simulink model "Scenario"  (Simulink 7.7)
settings: Solver=ode45  StartTime=0.0  StopTime=10.0  RelTol=1e-3
undefined symbols (not defined in the file): sigbuilder_block
libraries: simulink x4, instrumentlib x4, utility x1, dspnetwork x1
settings Model: Creator=Zsolt  LastModifiedBy=meta
settings HardwareCC: TargetIntDivRoundTo=Zero  TargetEndianess=LittleEndian  TargetHWDeviceType=MATLAB Host  ProdEqTarget=off
settings RTWCC: SystemTargetFile=rsim.tlc  TemplateMakefile=rsim_default_tmf  Description=Rapid Simulation Target  ProcessScript=rsim_make_rtw_hook
settings RSimTargetCC: TargetFunctionLibrary=ANSI_C  ERTMultiwordTypeDef=System defined  FunctionExecutionProfile=off  CodeExecutionProfiling=off  ERTCodeCoverageTool=None  ERTMultiwordLength=256  IsPILTarget=off  EnableShiftOperators=on  PortableWordSizes=off

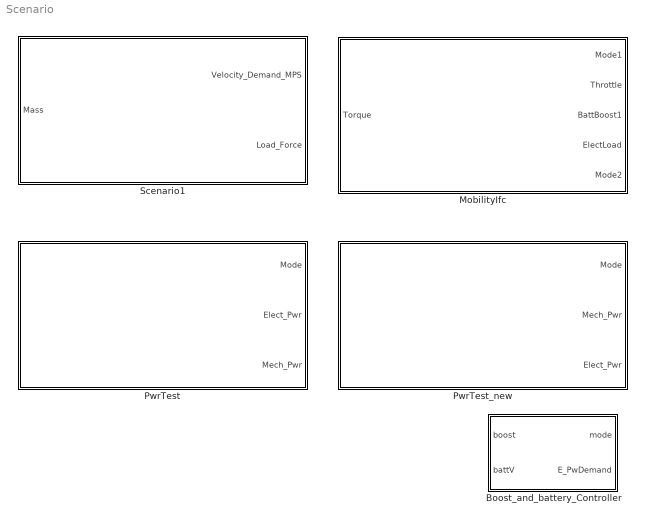
== system Scenario ==
  Boost_and_battery_Controller : Stateflow chart  TreatAsAtomicUnit=on
  MobilityIfc : Subsystem
  PwrTest : Subsystem
  PwrTest_new : Subsystem
  Scenario1 : Subsystem

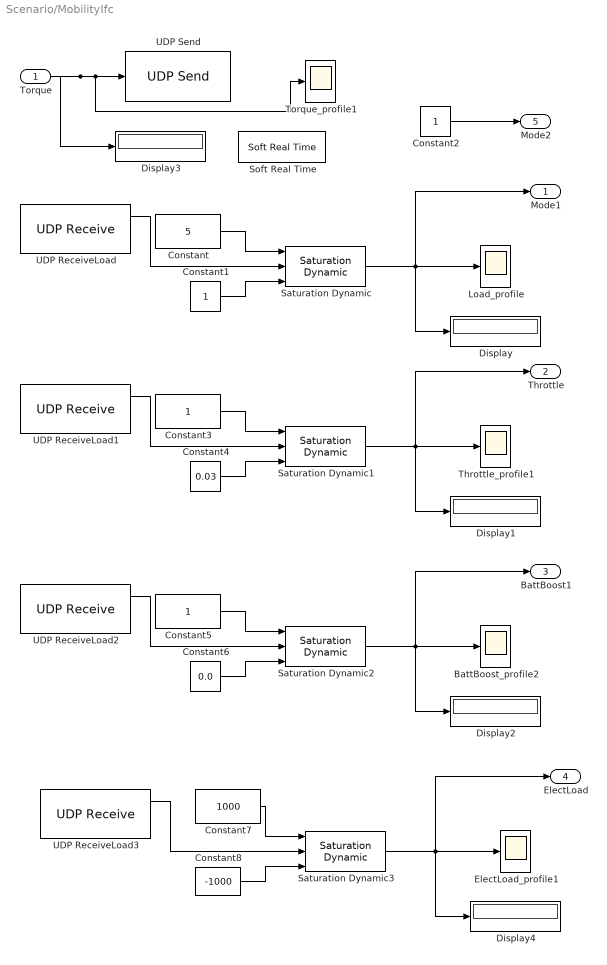
== system Scenario/MobilityIfc ==
  Torque : Inport
  BattBoost_profile2 : Scope
      settings: TimeRange=500  YMin=0  YMax=150000  SaveName=ScopeData3
  Constant : Constant  Value=5
  Constant{1..3,5} (4 alike) : Constant
  Constant4 : Constant  Value=0.03
  Constant6 : Constant  Value=0.0
  Constant7 : Constant  Value=1000
  Constant8 : Constant  Value=-1000
  Display{,1..4} (5 alike) : Display
  ElectLoad_profile1 : Scope
      settings: TimeRange=500  YMin=0  YMax=150000  SaveName=ScopeData5
  Load_profile : Scope
      settings: TimeRange=500  YMin=0  YMax=150000
  Saturation Dynamic{,1..3} (4 alike) : simulink/Discontinuities/Saturation Dynamic  SystemSampleTime=-1  OutMin=[]  OutMax=[]  OutDataTypeStr=Inherit: Same as second input  OutDataType=fixdt(1, 16)  OutScaling=2^-10  DoSatur=off
  Soft Real Time : utility/Soft Real Time  x=1
  Throttle_profile1 : Scope
      settings: TimeRange=500  YMin=0  YMax=150000
  Torque_profile1 : Scope
      settings: TimeRange=100  YMin=0  YMax=150000  SaveName=ScopeData4
  UDP ReceiveLoad : instrumentlib/UDP Receive  Host=localhost  Port=9090  LocalPort=8090  DataSize=[1 1]  EnableBlockingMode=off  Timeout=10  SampleTime=0.08  DataType=double  ByteOrder=LittleEndian
  UDP ReceiveLoad1 : instrumentlib/UDP Receive  Host=localhost  Port=9090  LocalPort=8092  DataSize=[1 1]  EnableBlockingMode=off  Timeout=10  SampleTime=0.08  DataType=double  ByteOrder=LittleEndian
  UDP ReceiveLoad2 : instrumentlib/UDP Receive  Host=localhost  Port=9090  LocalPort=8093  DataSize=[1 1]  EnableBlockingMode=off  Timeout=10  SampleTime=0.08  DataType=double  ByteOrder=LittleEndian
  UDP ReceiveLoad3 : instrumentlib/UDP Receive  Host=localhost  Port=9090  LocalPort=8098  DataSize=[1 1]  EnableBlockingMode=off  Timeout=10  SampleTime=0.08  DataType=double  ByteOrder=LittleEndian
  UDP Send : dspnetwork/UDP Send  remoteURL='127.0.0.1'  remotePort=8094  localURL='0.0.0.0'  localPortSource=Automatically determine  localPort=-1  sampletime=-1  separateLengthPort=0
  Mode1 : Outport
  Throttle : Outport  Port=2
  BattBoost1 : Outport  Port=3
  ElectLoad : Outport  Port=4
  Mode2 : Outport  Port=5
  wires:
  Constant/1 -> Saturation Dynamic/1
  Constant1/1 -> Saturation Dynamic/3
  Saturation Dynamic/1 -> Load_profile/1, Display/1, Mode1/1
  UDP ReceiveLoad/1 -> Saturation Dynamic/2
  Constant2/1 -> Mode2/1
  Constant3/1 -> Saturation Dynamic1/1
  Constant4/1 -> Saturation Dynamic1/3
  Saturation Dynamic1/1 -> Throttle_profile1/1, Display1/1, Throttle/1
  UDP ReceiveLoad1/1 -> Saturation Dynamic1/2
  Constant5/1 -> Saturation Dynamic2/1
  Constant6/1 -> Saturation Dynamic2/3
  Saturation Dynamic2/1 -> BattBoost_profile2/1, Display2/1, BattBoost1/1
  UDP ReceiveLoad2/1 -> Saturation Dynamic2/2
  Torque/1 -> UDP Send/1, Torque_profile1/1, Display3/1
  Constant7/1 -> Saturation Dynamic3/1
  Constant8/1 -> Saturation Dynamic3/3
  Saturation Dynamic3/1 -> ElectLoad_profile1/1, Display4/1, ElectLoad/1
  UDP ReceiveLoad3/1 -> Saturation Dynamic3/2

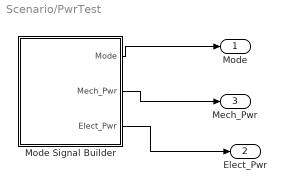
== system Scenario/PwrTest ==
  Mode Signal Builder : Subsystem  Tag=STV Subsys  LoadFcn=sigbuilder_block('load');  StartFcn=sigbuilder_block('start');  StopFcn=sigbuilder_block('stop');  ClipboardFcn=sigbuilder_block('clipboard');  mask(Sigbuilder block){}
      mask help: Create and generate interchangeable groups of signals whose waveforms are piecewise linear.
      mask init:
      | if ~strcmp(get_param(bdroot(gcbh),'SimulationStatus'),'stopped') tuvar = sigbuilder_block('maskInit'); end
      settings: CopyFcn=sigbuilder_block('copy');  DeleteFcn=sigbuilder_block('delete');  ModelCloseFcn=sigbuilder_block('modelClose');  PreSaveFcn=sigbuilder_block('preSave');  NameChangeFcn=sigbuilder_block('namechange');  OpenFcn=sigbuilder_block('open',[215.25 65.25 852.75 489.75 ]);  CloseFcn=sigbuilder_block('close');
      mask Display: plot(0,0,100,100,[10,10,40,40,10],[80,20,20,80,80],[40,10],[50,50], [40,27,10],[65,72,56],[40,25,25,10],[28,28,43,43]);
  Mode : Outport
  Elect_Pwr : Outport  Port=2
  Mech_Pwr : Outport  Port=3
  wires:
  Mode Signal Builder/1(Mode) -> Mode/1
  Mode Signal Builder/2(Mech_Pwr) -> Mech_Pwr/1
  Mode Signal Builder/3(Elect_Pwr) -> Elect_Pwr/1

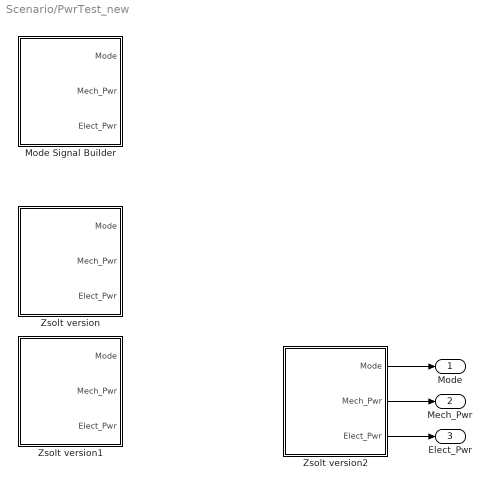
== system Scenario/PwrTest_new ==
  Mode Signal Builder : Subsystem  Tag=STV Subsys  LoadFcn=sigbuilder_block('load');  StartFcn=sigbuilder_block('start');  StopFcn=sigbuilder_block('stop');  ClipboardFcn=sigbuilder_block('clipboard');  mask(Sigbuilder block){}
      mask help: Create and generate interchangeable groups of signals whose waveforms are piecewise linear.
      mask init:
      | if ~strcmp(get_param(bdroot(gcbh),'SimulationStatus'),'stopped') tuvar = sigbuilder_block('maskInit'); end
      settings: CopyFcn=sigbuilder_block('copy');  DeleteFcn=sigbuilder_block('delete');  ModelCloseFcn=sigbuilder_block('modelClose');  PreSaveFcn=sigbuilder_block('preSave');  NameChangeFcn=sigbuilder_block('namechange');  OpenFcn=sigbuilder_block('open',[215.25 65.25 852.75 489.75 ]);  CloseFcn=sigbuilder_block('close');
      mask Display: plot(0,0,100,100,[10,10,40,40,10],[80,20,20,80,80],[40,10],[50,50], [40,27,10],[65,72,56],[40,25,25,10],[28,28,43,43]);
  Zsolt version : Subsystem  Tag=STV Subsys  LoadFcn=sigbuilder_block('load');  StartFcn=sigbuilder_block('start');  StopFcn=sigbuilder_block('stop');  ClipboardFcn=sigbuilder_block('clipboard');  mask(Sigbuilder block){}
      mask help: Create and generate interchangeable groups of signals whose waveforms are piecewise linear.
      mask init:
      | if ~strcmp(get_param(bdroot(gcbh),'SimulationStatus'),'stopped') tuvar = sigbuilder_block('maskInit'); end
      settings: CopyFcn=sigbuilder_block('copy');  DeleteFcn=sigbuilder_block('delete');  ModelCloseFcn=sigbuilder_block('modelClose');  PreSaveFcn=sigbuilder_block('preSave');  NameChangeFcn=sigbuilder_block('namechange');  OpenFcn=sigbuilder_block('open',[9 35.25 852.75 281.25 ]);  CloseFcn=sigbuilder_block('close');
      mask Display: plot(0,0,100,100,[10,10,40,40,10],[80,20,20,80,80],[40,10],[50,50], [40,27,10],[65,72,56],[40,25,25,10],[28,28,43,43]);
  Zsolt version1 : Subsystem  Tag=STV Subsys  LoadFcn=sigbuilder_block('load');  StartFcn=sigbuilder_block('start');  StopFcn=sigbuilder_block('stop');  ClipboardFcn=sigbuilder_block('clipboard');  mask(Sigbuilder block){}
      mask help: Create and generate interchangeable groups of signals whose waveforms are piecewise linear.
      mask init:
      | if ~strcmp(get_param(bdroot(gcbh),'SimulationStatus'),'stopped') tuvar = sigbuilder_block('maskInit'); end
      settings: CopyFcn=sigbuilder_block('copy');  DeleteFcn=sigbuilder_block('delete');  ModelCloseFcn=sigbuilder_block('modelClose');  PreSaveFcn=sigbuilder_block('preSave');  NameChangeFcn=sigbuilder_block('namechange');  OpenFcn=sigbuilder_block('open',[9 35.25 852.75 281.25 ]);  CloseFcn=sigbuilder_block('close');
      mask Display: plot(0,0,100,100,[10,10,40,40,10],[80,20,20,80,80],[40,10],[50,50], [40,27,10],[65,72,56],[40,25,25,10],[28,28,43,43]);
  Zsolt version2 : Subsystem  Tag=STV Subsys  LoadFcn=sigbuilder_block('load');  StartFcn=sigbuilder_block('start');  StopFcn=sigbuilder_block('stop');  ClipboardFcn=sigbuilder_block('clipboard');  mask(Sigbuilder block){}
      mask help: Create and generate interchangeable groups of signals whose waveforms are piecewise linear.
      mask init:
      | if ~strcmp(get_param(bdroot(gcbh),'SimulationStatus'),'stopped') tuvar = sigbuilder_block('maskInit'); end
      settings: CopyFcn=sigbuilder_block('copy');  DeleteFcn=sigbuilder_block('delete');  ModelCloseFcn=sigbuilder_block('modelClose');  PreSaveFcn=sigbuilder_block('preSave');  NameChangeFcn=sigbuilder_block('namechange');  OpenFcn=sigbuilder_block('open',[8.25 -66 852.75 246 ]);  CloseFcn=sigbuilder_block('close');
      mask Display: plot(0,0,100,100,[10,10,40,40,10],[80,20,20,80,80],[40,10],[50,50], [40,27,10],[65,72,56],[40,25,25,10],[28,28,43,43]);
  Mode : Outport
  Mech_Pwr : Outport  Port=2
  Elect_Pwr : Outport  Port=3
  wires:
  Zsolt version2/1(Mode) -> Mode/1
  Zsolt version2/2(Mech_Pwr) -> Mech_Pwr/1
  Zsolt version2/3(Elect_Pwr) -> Elect_Pwr/1

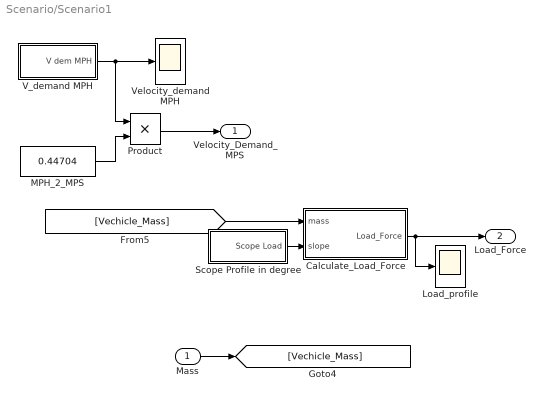
== system Scenario/Scenario1 ==
  Mass : Inport
  Calculate_Load_Force : Subsystem
  Load_profile : Scope
      settings: TimeRange=500  YMin=0  YMax=100000  SaveName=ScopeData7
  MPH_2_MPS : Constant  Value=0.44704
  Product : Product  RndMeth=Zero
  Scope Profile in degree : Subsystem  Tag=STV Subsys  LoadFcn=sigbuilder_block('load');  StartFcn=sigbuilder_block('start');  StopFcn=sigbuilder_block('stop');  ClipboardFcn=sigbuilder_block('clipboard');  mask(Sigbuilder block){}
      mask help: Create and generate interchangeable groups of signals whose waveforms are piecewise linear.
      mask init:
      | if ~strcmp(get_param(bdroot(gcbh),'SimulationStatus'),'stopped') tuvar = sigbuilder_block('maskInit'); end
      settings: CopyFcn=sigbuilder_block('copy');  DeleteFcn=sigbuilder_block('delete');  ModelCloseFcn=sigbuilder_block('modelClose');  PreSaveFcn=sigbuilder_block('preSave');  NameChangeFcn=sigbuilder_block('namechange');  OpenFcn=sigbuilder_block('open',[879 269.25 550.5 386.25 ]);  CloseFcn=sigbuilder_block('close');
      mask Display: plot(0,0,100,100,[10,10,40,40,10],[80,20,20,80,80],[40,10],[50,50], [40,27,10],[65,72,56],[40,25,25,10],[28,28,43,43]);
  V_demand MPH : Subsystem  Tag=STV Subsys  LoadFcn=sigbuilder_block('load');  StartFcn=sigbuilder_block('start');  StopFcn=sigbuilder_block('stop');  ClipboardFcn=sigbuilder_block('clipboard');  mask(Sigbuilder block){}
      mask help: Create and generate interchangeable groups of signals whose waveforms are piecewise linear.
      mask init:
      | if ~strcmp(get_param(bdroot(gcbh),'SimulationStatus'),'stopped') tuvar = sigbuilder_block('maskInit'); end
      settings: CopyFcn=sigbuilder_block('copy');  DeleteFcn=sigbuilder_block('delete');  ModelCloseFcn=sigbuilder_block('modelClose');  PreSaveFcn=sigbuilder_block('preSave');  NameChangeFcn=sigbuilder_block('namechange');  OpenFcn=sigbuilder_block('open',[827.25 153 606.75 301.5 ]);  CloseFcn=sigbuilder_block('close');
      mask Display: plot(0,0,100,100,[10,10,40,40,10],[80,20,20,80,80],[40,10],[50,50], [40,27,10],[65,72,56],[40,25,25,10],[28,28,43,43]);
  Velocity_demand MPH : Scope
      settings: TimeRange=500  YMin=0  YMax=60  SaveName=ScopeData2
  Velocity_Demand_MPS : Outport
  Load_Force : Outport  Port=2
  wires:
  MPH_2_MPS/1 -> Product/2
  V_demand MPH/1(V dem MPH) -> Product/1, Velocity_demand MPH/1
  Product/1 -> Velocity_Demand_MPS/1
  Calculate_Load_Force/1(Load_Force) -> Load_profile/1, Load_Force/1
  Scope Profile in degree/1(Scope Load) -> Calculate_Load_Force/2(slope)
  [Vechicle_Mass] -> Calculate_Load_Force/1(mass)
  Mass/1 -> [Vechicle_Mass]

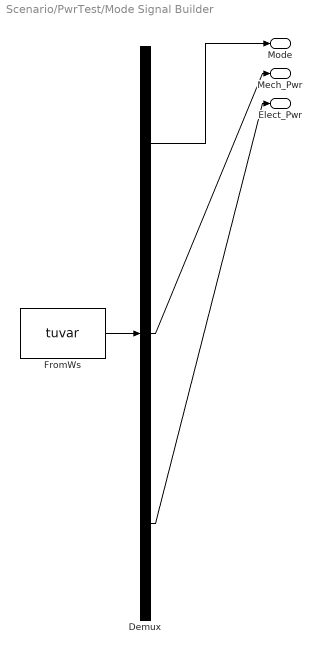
== system Scenario/PwrTest/Mode Signal Builder ==
  Demux : Demux  Tag=STV Demux  Outputs=3
  FromWs : FromWorkspace  Tag=STV FromWs  VariableName=tuvar  SampleTime=0  SigBuilderData=DataTag0  VnvData=DataTag1
      SigBuilderData=|
      | common.afterFinalStr = 'Extrapolate'
      | common.sampleTime = 0
      | dataSet.timeRange = [0 1000]
      | dataSet.name = 'Group 1'
      | sbobj.Groups.Name = 'Group 1'
      | sbobj.Groups.Signals(1).Name = 'Mode'
      | sbobj.Groups.Signals(1).XData = [0 62 62 398 1000]
      | sbobj.Groups.Signals(1).YData = [1 1 0 0 0]
      | sbobj.Groups.Signals(2).Name = 'Mech_Pwr'
      | sbobj.Groups.Signals(2).XData = [0 16 16 239 239 1000]
      | sbobj.Groups.Signals(2).YData = [0.58 0.58 0.24 0.24 0.44 0.44]
      | sbobj.Groups.Signals(3).Name = 'Elect_Pwr'
      | sbobj.Groups.Signals(3).XData = [0 16 16 44 44 60 60 81 81 1000]
      | sbobj.Groups.Signals(3).YData = [37 37 -32.5 -32.5 -0.5 -0.5 -1 -1 -1 -1]
      | sbobj.Groups.TimeRange = [0 1000]
  Mode : Outport  Tag=STV Outport
  Mech_Pwr : Outport  Tag=STV Outport  Port=2
  Elect_Pwr : Outport  Tag=STV Outport  Port=3
  wires:
  Demux/1 -> Mode/1
  FromWs/1 -> Demux/1
  Demux/2 -> Mech_Pwr/1
  Demux/3 -> Elect_Pwr/1

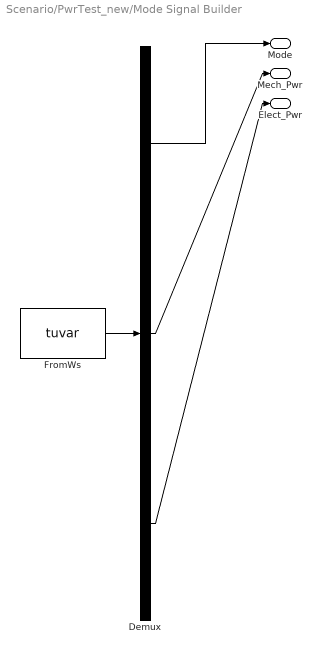
== system Scenario/PwrTest_new/Mode Signal Builder ==
  Demux : Demux  Tag=STV Demux  Outputs=3
  FromWs : FromWorkspace  Tag=STV FromWs  VariableName=tuvar  SampleTime=0  SigBuilderData=DataTag2  VnvData=DataTag3
      SigBuilderData=|
      | common.afterFinalStr = 'Extrapolate'
      | common.sampleTime = 0
      | dataSet.timeRange = [0 1000]
      | dataSet.name = 'Group 1'
      | sbobj.Groups.Name = 'Group 1'
      | sbobj.Groups.Signals(1).Name = 'Mode'
      | sbobj.Groups.Signals(1).XData = [0 62 62 398 1000]
      | sbobj.Groups.Signals(1).YData = [1 1 0 0 0]
      | sbobj.Groups.Signals(2).Name = 'Mech_Pwr'
      | sbobj.Groups.Signals(2).XData = [0 16 16 239 239 1000]
      | sbobj.Groups.Signals(2).YData = [0.58 0.58 0.24 0.24 0.44 0.44]
      | sbobj.Groups.Signals(3).Name = 'Elect_Pwr'
      | sbobj.Groups.Signals(3).XData = [0 16 16 44 44 60 60 81 81 1000]
      | sbobj.Groups.Signals(3).YData = [37 37 -32.5 -32.5 -0.5 -0.5 -1 -1 -1 -1]
      | sbobj.Groups.TimeRange = [0 1000]
  Mode : Outport  Tag=STV Outport
  Mech_Pwr : Outport  Tag=STV Outport  Port=2
  Elect_Pwr : Outport  Tag=STV Outport  Port=3
  wires:
  Demux/3 -> Elect_Pwr/1
  Demux/2 -> Mech_Pwr/1
  FromWs/1 -> Demux/1
  Demux/1 -> Mode/1

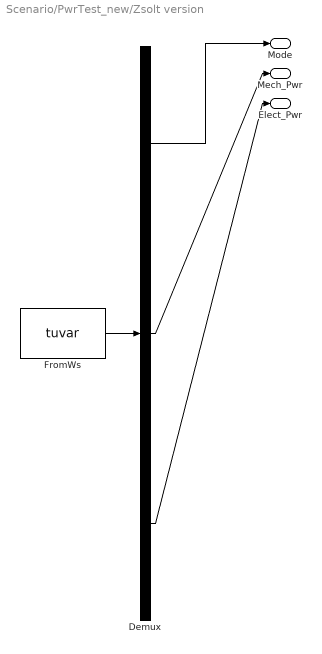
== system Scenario/PwrTest_new/Zsolt version ==
  Demux : Demux  Tag=STV Demux  Outputs=3
  FromWs : FromWorkspace  Tag=STV FromWs  VariableName=tuvar  SampleTime=0  SigBuilderData=DataTag4  VnvData=DataTag5
      SigBuilderData=|
      | common.afterFinalStr = 'Extrapolate'
      | common.sampleTime = 0
      | dataSet.timeRange = [0 100]
      | dataSet.name = 'Group 1'
      | sbobj.Groups.Name = 'Group 1'
      | sbobj.Groups.Signals(1).Name = 'Mode'
      | sbobj.Groups.Signals(1).XData = [0 62 62 100]
      | sbobj.Groups.Signals(1).YData = [1 1 0 0]
      | sbobj.Groups.Signals(2).Name = 'Mech_Pwr'
      | sbobj.Groups.Signals(2).XData = [0 24.7 100]
      | sbobj.Groups.Signals(2).YData = [0.68 0.68 0.24]
      | sbobj.Groups.Signals(3).Name = 'Elect_Pwr'
      | sbobj.Groups.Signals(3).XData = [0 2 2 25.6 25.6 28 28 100]
      | sbobj.Groups.Signals(3).YData = [-208 -208 -288 -284 -212 -212 -202 -202]
      | sbobj.Groups.TimeRange = [0 100]
  Mode : Outport  Tag=STV Outport
  Mech_Pwr : Outport  Tag=STV Outport  Port=2
  Elect_Pwr : Outport  Tag=STV Outport  Port=3
  wires:
  Demux/3 -> Elect_Pwr/1
  Demux/2 -> Mech_Pwr/1
  FromWs/1 -> Demux/1
  Demux/1 -> Mode/1

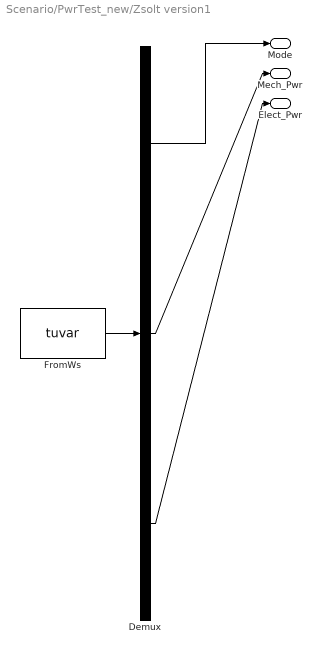
== system Scenario/PwrTest_new/Zsolt version1 ==
  Demux : Demux  Tag=STV Demux  Outputs=3
  FromWs : FromWorkspace  Tag=STV FromWs  VariableName=tuvar  SampleTime=0  SigBuilderData=DataTag6  VnvData=DataTag7
      SigBuilderData=|
      | common.afterFinalStr = 'Extrapolate'
      | common.sampleTime = 0
      | dataSet.timeRange = [0 100]
      | dataSet.name = 'Group 1'
      | sbobj.Groups.Name = 'Group 1'
      | sbobj.Groups.Signals(1).Name = 'Mode'
      | sbobj.Groups.Signals(1).XData = [0 27.2 27.2 100]
      | sbobj.Groups.Signals(1).YData = [1 1 0 0]
      | sbobj.Groups.Signals(2).Name = 'Mech_Pwr'
      | sbobj.Groups.Signals(2).XData = [0 24.7 24.7 100]
      | sbobj.Groups.Signals(2).YData = [1 1 0.99 0.99]
      | sbobj.Groups.Signals(3).Name = 'Elect_Pwr'
      | sbobj.Groups.Signals(3).XData = [0 7 7 11.8 11.8 28 28 100]
      | sbobj.Groups.Signals(3).YData = [5.5 5.5 -995 -995 5.5 5.5 -202 -202]
      | sbobj.Groups.TimeRange = [0 100]
  Mode : Outport  Tag=STV Outport
  Mech_Pwr : Outport  Tag=STV Outport  Port=2
  Elect_Pwr : Outport  Tag=STV Outport  Port=3
  wires:
  Demux/1 -> Mode/1
  FromWs/1 -> Demux/1
  Demux/2 -> Mech_Pwr/1
  Demux/3 -> Elect_Pwr/1

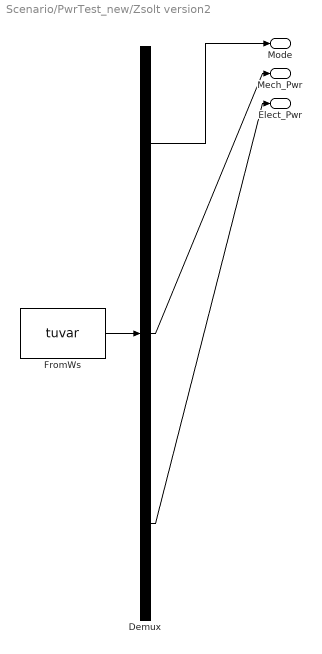
== system Scenario/PwrTest_new/Zsolt version2 ==
  Demux : Demux  Tag=STV Demux  Outputs=3
  FromWs : FromWorkspace  Tag=STV FromWs  VariableName=tuvar  SampleTime=0  SigBuilderData=DataTag8  VnvData=DataTag9
      SigBuilderData=|
      | common.afterFinalStr = 'Extrapolate'
      | common.sampleTime = 0
      | dataSet.timeRange = [0 100]
      | dataSet.name = 'Group 1'
      | sbobj.Groups.Name = 'Group 1'
      | sbobj.Groups.Signals(1).Name = 'Mode'
      | sbobj.Groups.Signals(1).XData = [0 19 19 90.2 100]
      | sbobj.Groups.Signals(1).YData = [0 0 1 1 1]
      | sbobj.Groups.Signals(2).Name = 'Mech_Pwr'
      | sbobj.Groups.Signals(2).XData = [0 72.2 72.2 100]
      | sbobj.Groups.Signals(2).YData = [1 1 0.58 0.58]
      | sbobj.Groups.Signals(3).Name = 'Elect_Pwr'
      | sbobj.Groups.Signals(3).XData = [0 36.1 36.1 44.8 44.8 52.9 52.9 100]
      | sbobj.Groups.Signals(3).YData = [20 20 -215 -215 -235 -235 5 5]
      | sbobj.Groups.TimeRange = [0 100]
  Mode : Outport  Tag=STV Outport
  Mech_Pwr : Outport  Tag=STV Outport  Port=2
  Elect_Pwr : Outport  Tag=STV Outport  Port=3
  wires:
  Demux/3 -> Elect_Pwr/1
  Demux/2 -> Mech_Pwr/1
  FromWs/1 -> Demux/1
  Demux/1 -> Mode/1

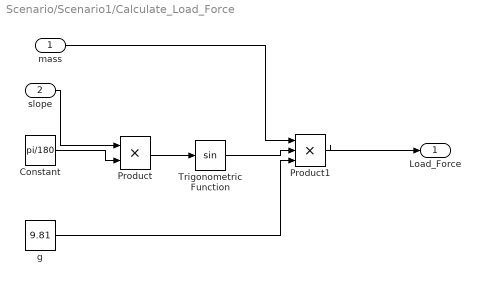
== system Scenario/Scenario1/Calculate_Load_Force ==
  mass : Inport
  slope : Inport  Port=2
  Constant : Constant  Value=pi/180
  Product : Product  RndMeth=Zero
  Product1 : Product  Inputs=3  RndMeth=Zero
  Trigonometric Function : Trigonometry
  g : Constant  Value=9.81
  Load_Force : Outport
  wires:
  Trigonometric Function/1 -> Product1/2
  Product/1 -> Trigonometric Function/1
  Constant/1 -> Product/2
  mass/1 -> Product1/1
  slope/1 -> Product/1
  Product1/1 -> Load_Force/1
  g/1 -> Product1/3

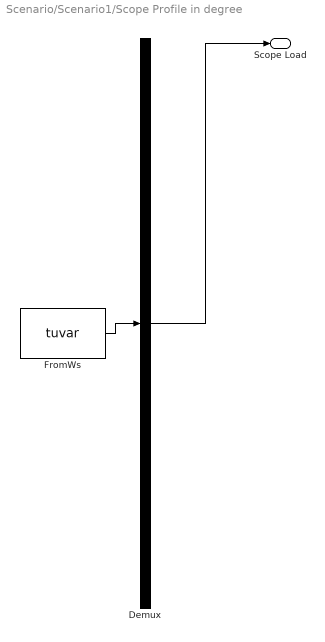
== system Scenario/Scenario1/Scope Profile in degree ==
  Demux : Demux  Tag=STV Demux  Outputs=1
  FromWs : FromWorkspace  Tag=STV FromWs  VariableName=tuvar  SampleTime=0  SigBuilderData=DataTag10  VnvData=DataTag11
      SigBuilderData=|
      | common.afterFinalStr = 'Extrapolate'
      | common.sampleTime = 0
      | dataSet.timeRange = [0 300]
      | dataSet.name = 'Group 1'
      | sbobj.Groups.Name = 'Group 1'
      | sbobj.Groups.Signals.Name = 'Scope Load'
      | sbobj.Groups.Signals.XData = [0 150.5 150.5 250.5 250.5 300]
      | sbobj.Groups.Signals.YData = [0 0 10 10 0 0]
      | sbobj.Groups.TimeRange = [0 300]
  Scope Load : Outport  Tag=STV Outport
  wires:
  Demux/1 -> Scope Load/1
  FromWs/1 -> Demux/1

== system Scenario/Scenario1/V_demand MPH ==
  Demux : Demux  Tag=STV Demux  Outputs=1
  FromWs : FromWorkspace  Tag=STV FromWs  VariableName=tuvar  SampleTime=0  SigBuilderData=DataTag12  VnvData=DataTag13
      SigBuilderData=|
      | common.afterFinalStr = 'Extrapolate'
      | common.sampleTime = 0
      | dataSet.timeRange = [0 300]
      | dataSet.name = 'Group 1'
      | sbobj.Groups.Name = 'Group 1'
      | sbobj.Groups.Signals.Name = 'V dem MPH'
      | sbobj.Groups.Signals.XData = [0 50 150 150 250 250 300]
      | sbobj.Groups.Signals.YData = [50 50 50 17 17 50 50]
      | sbobj.Groups.TimeRange = [0 300]
  V dem MPH : Outport  Tag=STV Outport
  wires:
  Demux/1 -> V dem MPH/1
  FromWs/1 -> Demux/1

== matlab function Boost_and_battery_Controller ==
  data: boost input double; mode output double; E_PwDemand output double; battV input double
function [mode, E_PwDemand] = fcn(boost, battV)
%#eml
%MaxBatteryV = 225;
BatteryMaxCharge = 210;
BatteryCritical = 185;
E_PwDemand_chg = 5.5;
E_PwDemand = E_PwDemand_chg;
mode = 0;
if (boost == 0)
  if (battV < BatteryMaxCharge)
    % charge
    E_PwDemand = E_PwDemand_chg;
    mode = 1;
  else
    % disconnect
    E_PwDemand = E_PwDemand_chg;
    mode = 0;
  end
elseif (battV > BatteryCritical)
  % use boost / discharge
  mode = boost;
  E_PwDemand = -BatteryMaxCharge;
end
%mode=1;
%E_PwDemand = -200;
